simulink model "exp4M_CSVPosRefCtrl"  (R2020a)
settings: Solver=FixedStepAuto  StartTime=0.0  StopTime=20.0313  RelTol=1e-3
InitFcn:
  | %Motor1 = Epos4(1,0);
  | %Motor2 = Epos4(2,0);
  | load exp2MSetup sm_path1
model workspace (MAT data in the model file):
  Kd1 = 0
  Kd2 = 0
  Kd3 = 0
  Kd4 = 0
  Ki1 = 7.10897656468
  Ki2 = 7.11405369329
  Ki3 = 7.10867391424
  Ki4 = 7.10556368704
  Kp1 = 103.345225154
  Kp2 = 107.682383041
  Kp3 = 112.167183406
  Kp4 = 116.854342442
  N1 = 100
  N2 = 100
  N3 = 100
  N4 = 100
undefined symbols (not defined in the file or in its folder): x28_000006_reduction, x607325_PPR
libraries: simulink x4
CloseFcn:
  | %delete(Motor1);
  | %delete(Motor2);
settings Model: DataDictionary=MotorInfo.sldd  SimulationMode=accelerator  EnablePacing=on  OrderedModelArguments=off  Creator=khoi  LastModifiedBy=khoi
settings DataIOCC: InspectSignalLogs=on
settings RTWCC: GenCodeOnly=on

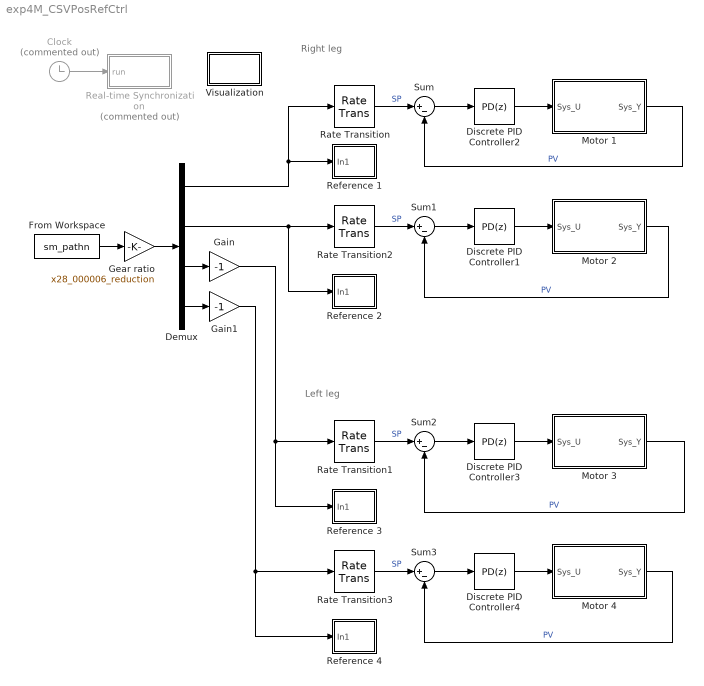
== system exp4M_CSVPosRefCtrl ==
  note: Right leg
  note: Left leg
  Clock : Clock  Commented=on
  Demux : Demux
  Discrete PID Controller1 : simulink/Continuous/PID Controller  Controller=PD  Form=Parallel  TimeDomain=Discrete-time  UseExternalTs=off  SampleTime=-1  IntegratorMethod=Forward Euler  FilterMethod=Forward Euler  ControllerParametersSource=internal  P=Kp2  I=Ki2  D=Kd2  UseFilter=on  N=N2  TunerSelectOption=Transfer Function Based (PID Tuner App)  InitialConditionSource=internal  InitialConditionForIntegrator=0  InitialConditionForFilter=0  DifferentiatorICPrevScaledInput=0  ExternalReset=none  TrackingMode=off  Kt=1  LimitOutput=off  UpperSaturationLimit=2000  LowerSaturationLimit=-2000  LinearizeAsGain=off  AntiWindupMode=clamping  Kb=1  POutMin=[]  POutMax=[]  IOutMin=[]  IOutMax=[]  DOutMin=[]  DOutMax=[]  NOutMin=[]  NOutMax=[]  SumOutMin=[]  SumOutMax=[]  SaturationOutMin=[]  SaturationOutMax=[]  PParamMin=[]  PParamMax=[]  IParamMin=[]  IParamMax=[]  DParamMin=[]  DParamMax=[]  NParamMin=[]  NParamMax=[]  KbParamMin=[]  KbParamMax=[]  KtParamMin=[]  KtParamMax=[]  KbOutMin=[]  KbOutMax=[]  KtOutMin=[]  KtOutMax=[]  IntegratorOutMin=[]  IntegratorOutMax=[]  FilterOutMin=[]  FilterOutMax=[]  SumI1OutMin=[]  SumI1OutMax=[]  SumI2OutMin=[]  SumI2OutMax=[]  SumI3OutMin=[]  SumI3OutMax=[]  SumI4OutMin=[]  SumI4OutMax=[]  SumDOutMin=[]  SumDOutMax=[]  DifferentiatorOutMin=[]  DifferentiatorOutMax=[]  FilterDiffOutCoefMin=[]  FilterDiffOutCoefMax=[]  ReciprocalOutMin=[]  ReciprocalOutMax=[]  SumDenOutMin=[]  SumDenOutMax=[]  SumNumOutMin=[]  SumNumOutMax=[]  DivideOutMin=[]  DivideOutMax=[]  UdiffTsProdOutMin=[]  UdiffTsProdOutMax=[]  NTsProdOutMin=[]  NTsProdOutMax=[]  UintegralTsProdOutMin=[]  UintegralTsProdOutMax=[]  UngainTsProdOutMin=[]  UngainTsProdOutMax=[]  IntegratorContinuousStateAttributes=''  IntegratorStateMustResolveToSignalObject=off  IntegratorRTWStateStorageClass=Auto  FilterContinuousStateAttributes=''  FilterStateMustResolveToSignalObject=off  FilterRTWStateStorageClass=Auto  ParallelPVariant=InternalParameters  IdealPVariant=Disabled  IVariant=Disabled  DVariant=InternalParameters  IntegratorVariant=Disabled  SatVariant=Disabled  AWVariant=Disabled  PCopyVariant=Disabled  TRVariant=Disabled  FdbkBlocksVariant=Forward  IdealPFdbkVariant=Disabled  SatFdbkVariant=Disabled  DerivativeFilterVariant=ForwardEulerFilter  NVariant=InternalParameters  NCopyVariant=Disabled  FilterICVariant=InternalICsFilter  IntegratorICVariant=Disabled  ExternalResetVariant=Disabled  TRSumVariant=Passthrough  SumFdbkVariant=Disabled  SumVariant=Sum_PD  TsampFilterVariant=InternalTs  TsampNgainVariant=Passthrough  TsampIntegralVariant=Disabled_SignalSpec
  Discrete PID Controller2 : simulink/Continuous/PID Controller  Controller=PD  Form=Parallel  TimeDomain=Discrete-time  UseExternalTs=off  SampleTime=-1  IntegratorMethod=Forward Euler  FilterMethod=Forward Euler  ControllerParametersSource=internal  P=Kp1  I=Ki1  D=Kd1  UseFilter=on  N=N1  TunerSelectOption=Transfer Function Based (PID Tuner App)  InitialConditionSource=internal  InitialConditionForIntegrator=0  InitialConditionForFilter=0  DifferentiatorICPrevScaledInput=0  ExternalReset=none  TrackingMode=off  Kt=1  LimitOutput=off  UpperSaturationLimit=2000  LowerSaturationLimit=-2000  LinearizeAsGain=off  AntiWindupMode=clamping  Kb=1  POutMin=[]  POutMax=[]  IOutMin=[]  IOutMax=[]  DOutMin=[]  DOutMax=[]  NOutMin=[]  NOutMax=[]  SumOutMin=[]  SumOutMax=[]  SaturationOutMin=[]  SaturationOutMax=[]  PParamMin=[]  PParamMax=[]  IParamMin=[]  IParamMax=[]  DParamMin=[]  DParamMax=[]  NParamMin=[]  NParamMax=[]  KbParamMin=[]  KbParamMax=[]  KtParamMin=[]  KtParamMax=[]  KbOutMin=[]  KbOutMax=[]  KtOutMin=[]  KtOutMax=[]  IntegratorOutMin=[]  IntegratorOutMax=[]  FilterOutMin=[]  FilterOutMax=[]  SumI1OutMin=[]  SumI1OutMax=[]  SumI2OutMin=[]  SumI2OutMax=[]  SumI3OutMin=[]  SumI3OutMax=[]  SumI4OutMin=[]  SumI4OutMax=[]  SumDOutMin=[]  SumDOutMax=[]  DifferentiatorOutMin=[]  DifferentiatorOutMax=[]  FilterDiffOutCoefMin=[]  FilterDiffOutCoefMax=[]  ReciprocalOutMin=[]  ReciprocalOutMax=[]  SumDenOutMin=[]  SumDenOutMax=[]  SumNumOutMin=[]  SumNumOutMax=[]  DivideOutMin=[]  DivideOutMax=[]  UdiffTsProdOutMin=[]  UdiffTsProdOutMax=[]  NTsProdOutMin=[]  NTsProdOutMax=[]  UintegralTsProdOutMin=[]  UintegralTsProdOutMax=[]  UngainTsProdOutMin=[]  UngainTsProdOutMax=[]  IntegratorContinuousStateAttributes=''  IntegratorStateMustResolveToSignalObject=off  IntegratorRTWStateStorageClass=Auto  FilterContinuousStateAttributes=''  FilterStateMustResolveToSignalObject=off  FilterRTWStateStorageClass=Auto  ParallelPVariant=InternalParameters  IdealPVariant=Disabled  IVariant=Disabled  DVariant=InternalParameters  IntegratorVariant=Disabled  SatVariant=Disabled  AWVariant=Disabled  PCopyVariant=Disabled  TRVariant=Disabled  FdbkBlocksVariant=Forward  IdealPFdbkVariant=Disabled  SatFdbkVariant=Disabled  DerivativeFilterVariant=ForwardEulerFilter  NVariant=InternalParameters  NCopyVariant=Disabled  FilterICVariant=InternalICsFilter  IntegratorICVariant=Disabled  ExternalResetVariant=Disabled  TRSumVariant=Passthrough  SumFdbkVariant=Disabled  SumVariant=Sum_PD  TsampFilterVariant=InternalTs  TsampNgainVariant=Passthrough  TsampIntegralVariant=Disabled_SignalSpec
  Discrete PID Controller3 : simulink/Continuous/PID Controller  Controller=PD  Form=Parallel  TimeDomain=Discrete-time  UseExternalTs=off  SampleTime=-1  IntegratorMethod=Forward Euler  FilterMethod=Forward Euler  ControllerParametersSource=internal  P=Kp3  I=Ki3  D=Kd3  UseFilter=on  N=N3  TunerSelectOption=Transfer Function Based (PID Tuner App)  InitialConditionSource=internal  InitialConditionForIntegrator=0  InitialConditionForFilter=0  DifferentiatorICPrevScaledInput=0  ExternalReset=none  TrackingMode=off  Kt=1  LimitOutput=off  UpperSaturationLimit=2000  LowerSaturationLimit=-2000  LinearizeAsGain=off  AntiWindupMode=clamping  Kb=1  POutMin=[]  POutMax=[]  IOutMin=[]  IOutMax=[]  DOutMin=[]  DOutMax=[]  NOutMin=[]  NOutMax=[]  SumOutMin=[]  SumOutMax=[]  SaturationOutMin=[]  SaturationOutMax=[]  PParamMin=[]  PParamMax=[]  IParamMin=[]  IParamMax=[]  DParamMin=[]  DParamMax=[]  NParamMin=[]  NParamMax=[]  KbParamMin=[]  KbParamMax=[]  KtParamMin=[]  KtParamMax=[]  KbOutMin=[]  KbOutMax=[]  KtOutMin=[]  KtOutMax=[]  IntegratorOutMin=[]  IntegratorOutMax=[]  FilterOutMin=[]  FilterOutMax=[]  SumI1OutMin=[]  SumI1OutMax=[]  SumI2OutMin=[]  SumI2OutMax=[]  SumI3OutMin=[]  SumI3OutMax=[]  SumI4OutMin=[]  SumI4OutMax=[]  SumDOutMin=[]  SumDOutMax=[]  DifferentiatorOutMin=[]  DifferentiatorOutMax=[]  FilterDiffOutCoefMin=[]  FilterDiffOutCoefMax=[]  ReciprocalOutMin=[]  ReciprocalOutMax=[]  SumDenOutMin=[]  SumDenOutMax=[]  SumNumOutMin=[]  SumNumOutMax=[]  DivideOutMin=[]  DivideOutMax=[]  UdiffTsProdOutMin=[]  UdiffTsProdOutMax=[]  NTsProdOutMin=[]  NTsProdOutMax=[]  UintegralTsProdOutMin=[]  UintegralTsProdOutMax=[]  UngainTsProdOutMin=[]  UngainTsProdOutMax=[]  IntegratorContinuousStateAttributes=''  IntegratorStateMustResolveToSignalObject=off  IntegratorRTWStateStorageClass=Auto  FilterContinuousStateAttributes=''  FilterStateMustResolveToSignalObject=off  FilterRTWStateStorageClass=Auto  ParallelPVariant=InternalParameters  IdealPVariant=Disabled  IVariant=Disabled  DVariant=InternalParameters  IntegratorVariant=Disabled  SatVariant=Disabled  AWVariant=Disabled  PCopyVariant=Disabled  TRVariant=Disabled  FdbkBlocksVariant=Forward  IdealPFdbkVariant=Disabled  SatFdbkVariant=Disabled  DerivativeFilterVariant=ForwardEulerFilter  NVariant=InternalParameters  NCopyVariant=Disabled  FilterICVariant=InternalICsFilter  IntegratorICVariant=Disabled  ExternalResetVariant=Disabled  TRSumVariant=Passthrough  SumFdbkVariant=Disabled  SumVariant=Sum_PD  TsampFilterVariant=InternalTs  TsampNgainVariant=Passthrough  TsampIntegralVariant=Disabled_SignalSpec
  Discrete PID Controller4 : simulink/Continuous/PID Controller  Controller=PD  Form=Parallel  TimeDomain=Discrete-time  UseExternalTs=off  SampleTime=-1  IntegratorMethod=Forward Euler  FilterMethod=Forward Euler  ControllerParametersSource=internal  P=Kp4  I=Ki4  D=Kd4  UseFilter=on  N=N4  TunerSelectOption=Transfer Function Based (PID Tuner App)  InitialConditionSource=internal  InitialConditionForIntegrator=0  InitialConditionForFilter=0  DifferentiatorICPrevScaledInput=0  ExternalReset=none  TrackingMode=off  Kt=1  LimitOutput=off  UpperSaturationLimit=2000  LowerSaturationLimit=-2000  LinearizeAsGain=off  AntiWindupMode=clamping  Kb=1  POutMin=[]  POutMax=[]  IOutMin=[]  IOutMax=[]  DOutMin=[]  DOutMax=[]  NOutMin=[]  NOutMax=[]  SumOutMin=[]  SumOutMax=[]  SaturationOutMin=[]  SaturationOutMax=[]  PParamMin=[]  PParamMax=[]  IParamMin=[]  IParamMax=[]  DParamMin=[]  DParamMax=[]  NParamMin=[]  NParamMax=[]  KbParamMin=[]  KbParamMax=[]  KtParamMin=[]  KtParamMax=[]  KbOutMin=[]  KbOutMax=[]  KtOutMin=[]  KtOutMax=[]  IntegratorOutMin=[]  IntegratorOutMax=[]  FilterOutMin=[]  FilterOutMax=[]  SumI1OutMin=[]  SumI1OutMax=[]  SumI2OutMin=[]  SumI2OutMax=[]  SumI3OutMin=[]  SumI3OutMax=[]  SumI4OutMin=[]  SumI4OutMax=[]  SumDOutMin=[]  SumDOutMax=[]  DifferentiatorOutMin=[]  DifferentiatorOutMax=[]  FilterDiffOutCoefMin=[]  FilterDiffOutCoefMax=[]  ReciprocalOutMin=[]  ReciprocalOutMax=[]  SumDenOutMin=[]  SumDenOutMax=[]  SumNumOutMin=[]  SumNumOutMax=[]  DivideOutMin=[]  DivideOutMax=[]  UdiffTsProdOutMin=[]  UdiffTsProdOutMax=[]  NTsProdOutMin=[]  NTsProdOutMax=[]  UintegralTsProdOutMin=[]  UintegralTsProdOutMax=[]  UngainTsProdOutMin=[]  UngainTsProdOutMax=[]  IntegratorContinuousStateAttributes=''  IntegratorStateMustResolveToSignalObject=off  IntegratorRTWStateStorageClass=Auto  FilterContinuousStateAttributes=''  FilterStateMustResolveToSignalObject=off  FilterRTWStateStorageClass=Auto  ParallelPVariant=InternalParameters  IdealPVariant=Disabled  IVariant=Disabled  DVariant=InternalParameters  IntegratorVariant=Disabled  SatVariant=Disabled  AWVariant=Disabled  PCopyVariant=Disabled  TRVariant=Disabled  FdbkBlocksVariant=Forward  IdealPFdbkVariant=Disabled  SatFdbkVariant=Disabled  DerivativeFilterVariant=ForwardEulerFilter  NVariant=InternalParameters  NCopyVariant=Disabled  FilterICVariant=InternalICsFilter  IntegratorICVariant=Disabled  ExternalResetVariant=Disabled  TRSumVariant=Passthrough  SumFdbkVariant=Disabled  SumVariant=Sum_PD  TsampFilterVariant=InternalTs  TsampNgainVariant=Passthrough  TsampIntegralVariant=Disabled_SignalSpec
  From Workspace : FromWorkspace  VariableName=sm_pathn  SampleTime=0.01
  Gain : Gain  Gain=-1
  Gain1 : Gain  Gain=-1
  Gear ratio : Gain  Gain=x28_000006_reduction
  Motor 1 : Subsystem
  Motor 2 : Subsystem
  Motor 3 : Subsystem
  Motor 4 : Subsystem
  Rate Transition{,1..3} (4 alike) : RateTransition  OutPortSampleTime=0.02
  Real-time Synchronization : Subsystem  Commented=on
  Reference 1 : Subsystem
  Reference 2 : Subsystem
  Reference 3 : Subsystem
  Reference 4 : Subsystem
  Sum{,1..3} (4 alike) : Sum  Inputs=|+-
  Visualization : Subsystem
  wires:
  Clock/1 -> Real-time Synchronization/1(run)
  Demux/1 -> Rate Transition/1, Reference 1/1(In1)
  Sum/1 -> Discrete PID Controller2/1
  Sum1/1 -> Discrete PID Controller1/1
  From Workspace/1 -> Gear ratio/1
  Demux/2 -> Reference 2/1(In1), Rate Transition2/1
  Gear ratio/1 -> Demux/1
  Rate Transition/1 -> Sum/1  "SP"
  Discrete PID Controller2/1 -> Motor 1/1(Sys_U)
  Motor 1/1(Sys_Y) -> Sum/2  "PV"
  Discrete PID Controller1/1 -> Motor 2/1(Sys_U)
  Rate Transition2/1 -> Sum1/1  "SP"
  Rate Transition1/1 -> Sum2/1  "SP"
  Motor 3/1(Sys_Y) -> Sum2/2  "PV"
  Discrete PID Controller3/1 -> Motor 3/1(Sys_U)
  Sum2/1 -> Discrete PID Controller3/1
  Sum3/1 -> Discrete PID Controller4/1
  Discrete PID Controller4/1 -> Motor 4/1(Sys_U)
  Motor 4/1(Sys_Y) -> Sum3/2  "PV"
  Rate Transition3/1 -> Sum3/1  "SP"
  Demux/3 -> Gain/1
  Demux/4 -> Gain1/1
  Gain/1 -> Rate Transition1/1, Reference 3/1(In1)
  Gain1/1 -> Reference 4/1(In1), Rate Transition3/1
  Motor 2/1(Sys_Y) -> Sum1/2  "PV"

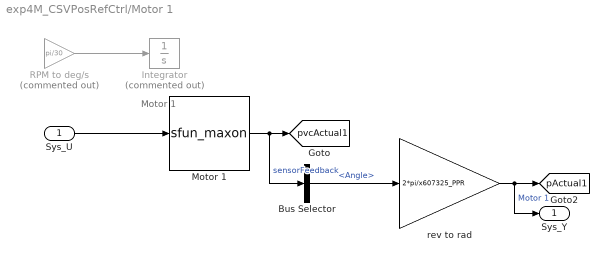
== system exp4M_CSVPosRefCtrl/Motor 1 ==
  note: Motor 1
  Sys_U : Inport
  Bus Selector : BusSelector  OutputSignals=Angle
  Integrator : Integrator  Commented=on
  Motor 1 : S-Function  FunctionName=sfun_maxon  Parameters=NodeID, DeltaT, OpMode  SFunctionDeploymentMode=off  EnableBusSupport=off  mask{NodeID=1, DeltaT=0.2, OpMode=Cyclic synchronous velocity mode, P_cur=0, I_cur=0, P_pos=0, I_pos=0, D_pos=0, v_posGainFF=0, a_posGainFF=0, P_vel=0, I_vel=0, v_velGainFF=0, a_velGainFF=0, f_velCutoff=0}
      mask prompts: NodeID "Node ID"; DeltaT "Sample time (s)"; OpMode "Operation mode"; P_cur "P gain"; I_cur "I gain"; P_pos "P gain"; I_pos "I gain"; D_pos "D gain"; v_posGainFF "FF velocity gain"; a_posGainFF "FF acceleration gain"; P_vel "P gain"; I_vel "I gain"; v_velGainFF "Feed-forward velocity gain"; a_velGainFF "Feed-forward acceleration gain"; f_velCutoff "Filter cut-off frequency"
      mask TypeOptions OpMode: Cyclic synchronous current (torque) mode | Cyclic synchronous velocity mode | Cyclic synchronous position mode | Profile velocity mode | Profile position mode
      mask DialogControl DescGroupVar Prompt: Motor Parameters
      mask DialogControl DescTextVar Prompt: The block outputs MotorInfo bus signal, which consists of the following variables: angle (increment), speed (rpm), current (mA)
      mask DialogControl Container6 Prompt: Motor
      mask DialogControl Container14 Prompt: Controller Parameters
      mask DialogControl DescTextVar_copy Prompt: This tab is experimental and does not implemented yet. Changing these parameters will not affect the motor performance.
      mask DialogControl Container15 Prompt: Current controller parameter set
      mask DialogControl Container15_copy Prompt: Position controller parameter set
      mask DialogControl Container15_copy_copy Prompt: Velocity controller parameter set
      mask Display:
      | disp('Maxon motor\nHIL');
      | % port_label('input', 1, 'inputSignal');
      | % port_label('output', 1, 'SENSR');
  RPM to deg/s : Gain  Commented=on  Gain=pi/30
  rev to rad : Gain  Gain=2*pi/x607325_PPR
  Sys_Y : Outport
  tag scope: pActual1=global, pvcActual1=global
  wires:
  Motor 1/1 -> [pvcActual1], Bus Selector/1  "sensorFeedback"
  rev to rad/1 -> Sys_Y/1, [pActual1]  "Motor 1"
  Sys_U/1 -> Motor 1/1
  RPM to deg/s/1 -> Integrator/1
  Bus Selector/1 -> rev to rad/1  "<Angle>"

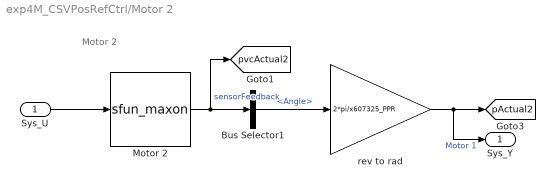
== system exp4M_CSVPosRefCtrl/Motor 2 ==
  note: Motor 2
  Sys_U : Inport
  Bus Selector1 : BusSelector  OutputSignals=Angle
  Motor 2 : S-Function  FunctionName=sfun_maxon  Parameters=NodeID, DeltaT, OpMode  SFunctionDeploymentMode=off  EnableBusSupport=off  mask{NodeID=2, DeltaT=0.2, OpMode=Cyclic synchronous velocity mode, P_cur=0, I_cur=0, P_pos=0, I_pos=0, D_pos=0, v_posGainFF=0, a_posGainFF=0, P_vel=0, I_vel=0, v_velGainFF=0, a_velGainFF=0, f_velCutoff=0}
      mask prompts: NodeID "Node ID"; DeltaT "Sample time (s)"; OpMode "Operation mode"; P_cur "P gain"; I_cur "I gain"; P_pos "P gain"; I_pos "I gain"; D_pos "D gain"; v_posGainFF "FF velocity gain"; a_posGainFF "FF acceleration gain"; P_vel "P gain"; I_vel "I gain"; v_velGainFF "Feed-forward velocity gain"; a_velGainFF "Feed-forward acceleration gain"; f_velCutoff "Filter cut-off frequency"
      mask TypeOptions OpMode: Cyclic synchronous current (torque) mode | Cyclic synchronous velocity mode | Cyclic synchronous position mode | Profile velocity mode | Profile position mode
      mask DialogControl DescGroupVar Prompt: Motor Parameters
      mask DialogControl DescTextVar Prompt: The block outputs MotorInfo bus signal, which consists of the following variables: angle (increment), speed (rpm), current (mA)
      mask DialogControl Container6 Prompt: Motor
      mask DialogControl Container14 Prompt: Controller Parameters
      mask DialogControl DescTextVar_copy Prompt: This tab is experimental and does not implemented yet. Changing these parameters will not affect the motor performance.
      mask DialogControl Container15 Prompt: Current controller parameter set
      mask DialogControl Container15_copy Prompt: Position controller parameter set
      mask DialogControl Container15_copy_copy Prompt: Velocity controller parameter set
      mask Display:
      | disp('Maxon motor\nHIL');
      | % port_label('input', 1, 'inputSignal');
      | % port_label('output', 1, 'SENSR');
  rev to rad : Gain  Gain=2*pi/x607325_PPR
  Sys_Y : Outport
  tag scope: pActual2=global, pvcActual2=global
  wires:
  Bus Selector1/1 -> rev to rad/1  "<Angle>"
  Sys_U/1 -> Motor 2/1
  rev to rad/1 -> Sys_Y/1, [pActual2]  "Motor 1"
  Motor 2/1 -> [pvcActual2], Bus Selector1/1  "sensorFeedback"

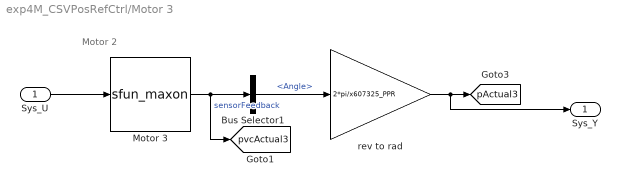
== system exp4M_CSVPosRefCtrl/Motor 3 ==
  note: Motor 2
  Sys_U : Inport
  Bus Selector1 : BusSelector  OutputSignals=Angle
  Motor 3 : S-Function  FunctionName=sfun_maxon  Parameters=NodeID, DeltaT, OpMode  SFunctionDeploymentMode=off  EnableBusSupport=off  mask{NodeID=3, DeltaT=0.2, OpMode=Cyclic synchronous velocity mode, P_cur=0, I_cur=0, P_pos=0, I_pos=0, D_pos=0, v_posGainFF=0, a_posGainFF=0, P_vel=0, I_vel=0, v_velGainFF=0, a_velGainFF=0, f_velCutoff=0}
      mask prompts: NodeID "Node ID"; DeltaT "Sample time (s)"; OpMode "Operation mode"; P_cur "P gain"; I_cur "I gain"; P_pos "P gain"; I_pos "I gain"; D_pos "D gain"; v_posGainFF "FF velocity gain"; a_posGainFF "FF acceleration gain"; P_vel "P gain"; I_vel "I gain"; v_velGainFF "Feed-forward velocity gain"; a_velGainFF "Feed-forward acceleration gain"; f_velCutoff "Filter cut-off frequency"
      mask TypeOptions OpMode: Cyclic synchronous current (torque) mode | Cyclic synchronous velocity mode | Cyclic synchronous position mode | Profile velocity mode | Profile position mode
      mask DialogControl DescGroupVar Prompt: Motor Parameters
      mask DialogControl DescTextVar Prompt: The block outputs MotorInfo bus signal, which consists of the following variables: angle (increment), speed (rpm), current (mA)
      mask DialogControl Container6 Prompt: Motor
      mask DialogControl Container14 Prompt: Controller Parameters
      mask DialogControl DescTextVar_copy Prompt: This tab is experimental and does not implemented yet. Changing these parameters will not affect the motor performance.
      mask DialogControl Container15 Prompt: Current controller parameter set
      mask DialogControl Container15_copy Prompt: Position controller parameter set
      mask DialogControl Container15_copy_copy Prompt: Velocity controller parameter set
      mask Display:
      | disp('Maxon motor\nHIL');
      | % port_label('input', 1, 'inputSignal');
      | % port_label('output', 1, 'SENSR');
  rev to rad : Gain  Gain=2*pi/x607325_PPR
  Sys_Y : Outport
  tag scope: pActual3=global, pvcActual3=global
  wires:
  Sys_U/1 -> Motor 3/1
  Bus Selector1/1 -> rev to rad/1  "<Angle>"
  rev to rad/1 -> Sys_Y/1, [pActual3]
  Motor 3/1 -> Bus Selector1/1, [pvcActual3]  "sensorFeedback"

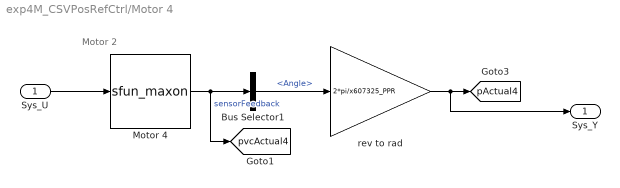
== system exp4M_CSVPosRefCtrl/Motor 4 ==
  note: Motor 2
  Sys_U : Inport
  Bus Selector1 : BusSelector  OutputSignals=Angle
  Motor 4 : S-Function  FunctionName=sfun_maxon  Parameters=NodeID, DeltaT, OpMode  SFunctionDeploymentMode=off  EnableBusSupport=off  mask{NodeID=4, DeltaT=0.2, OpMode=Cyclic synchronous velocity mode, P_cur=0, I_cur=0, P_pos=0, I_pos=0, D_pos=0, v_posGainFF=0, a_posGainFF=0, P_vel=0, I_vel=0, v_velGainFF=0, a_velGainFF=0, f_velCutoff=0}
      mask prompts: NodeID "Node ID"; DeltaT "Sample time (s)"; OpMode "Operation mode"; P_cur "P gain"; I_cur "I gain"; P_pos "P gain"; I_pos "I gain"; D_pos "D gain"; v_posGainFF "FF velocity gain"; a_posGainFF "FF acceleration gain"; P_vel "P gain"; I_vel "I gain"; v_velGainFF "Feed-forward velocity gain"; a_velGainFF "Feed-forward acceleration gain"; f_velCutoff "Filter cut-off frequency"
      mask TypeOptions OpMode: Cyclic synchronous current (torque) mode | Cyclic synchronous velocity mode | Cyclic synchronous position mode | Profile velocity mode | Profile position mode
      mask DialogControl DescGroupVar Prompt: Motor Parameters
      mask DialogControl DescTextVar Prompt: The block outputs MotorInfo bus signal, which consists of the following variables: angle (increment), speed (rpm), current (mA)
      mask DialogControl Container6 Prompt: Motor
      mask DialogControl Container14 Prompt: Controller Parameters
      mask DialogControl DescTextVar_copy Prompt: This tab is experimental and does not implemented yet. Changing these parameters will not affect the motor performance.
      mask DialogControl Container15 Prompt: Current controller parameter set
      mask DialogControl Container15_copy Prompt: Position controller parameter set
      mask DialogControl Container15_copy_copy Prompt: Velocity controller parameter set
      mask Display:
      | disp('Maxon motor\nHIL');
      | % port_label('input', 1, 'inputSignal');
      | % port_label('output', 1, 'SENSR');
  rev to rad : Gain  Gain=2*pi/x607325_PPR
  Sys_Y : Outport
  tag scope: pActual4=global, pvcActual4=global
  wires:
  Sys_U/1 -> Motor 4/1
  Bus Selector1/1 -> rev to rad/1  "<Angle>"
  rev to rad/1 -> Sys_Y/1, [pActual4]
  Motor 4/1 -> [pvcActual4], Bus Selector1/1  "sensorFeedback"

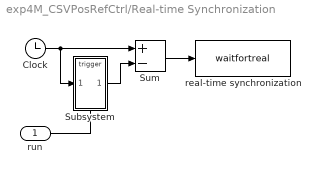
== system exp4M_CSVPosRefCtrl/Real-time Synchronization ==
  run : Inport
  Clock : Clock
  Subsystem : Subsystem  TreatAsAtomicUnit=on
  Sum : Sum  Inputs=+-  InputSameDT=on  SaturateOnIntegerOverflow=on  OutDataTypeStr=Inherit: Same as first input
  real-time synchronization : MATLABFcn  MATLABFcn=waitfortreal  OutputDimensions=0
  wires:
  Clock/1 -> Subsystem/1(In), Sum/1
  Subsystem/1(Out) -> Sum/2
  Sum/1 -> real-time synchronization/1
  run/1 -> Subsystem/Trigger

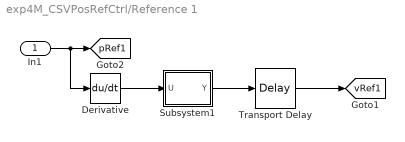
== system exp4M_CSVPosRefCtrl/Reference 1 ==
  In1 : Inport
  Derivative : Derivative
  Subsystem1 : Subsystem
      mask Display: disp('To rpm')
  Transport Delay : TransportDelay  DelayTime=0.1
  tag scope: pRef1=global, vRef1=global
  wires:
  Subsystem1/1(Y) -> Transport Delay/1
  Derivative/1 -> Subsystem1/1(U)
  In1/1 -> Derivative/1, [pRef1]
  Transport Delay/1 -> [vRef1]

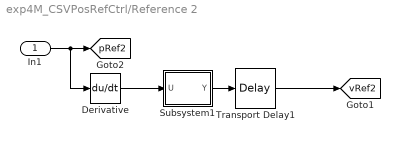
== system exp4M_CSVPosRefCtrl/Reference 2 ==
  In1 : Inport
  Derivative : Derivative
  Subsystem1 : Subsystem
      mask Display: disp('To rpm')
  Transport Delay1 : TransportDelay  DelayTime=0.1
  tag scope: pRef2=global, vRef2=global
  wires:
  Subsystem1/1(Y) -> Transport Delay1/1
  In1/1 -> [pRef2], Derivative/1
  Derivative/1 -> Subsystem1/1(U)
  Transport Delay1/1 -> [vRef2]

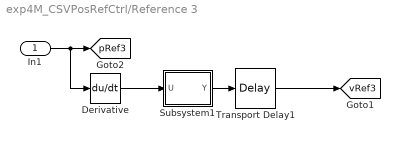
== system exp4M_CSVPosRefCtrl/Reference 3 ==
  In1 : Inport
  Derivative : Derivative
  Subsystem1 : Subsystem
      mask Display: disp('To rpm')
  Transport Delay1 : TransportDelay  DelayTime=0.1
  tag scope: pRef3=global, vRef3=global
  wires:
  Transport Delay1/1 -> [vRef3]
  Derivative/1 -> Subsystem1/1(U)
  In1/1 -> Derivative/1, [pRef3]
  Subsystem1/1(Y) -> Transport Delay1/1

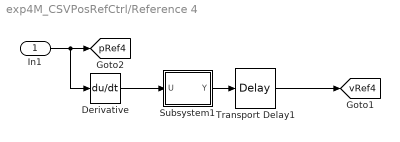
== system exp4M_CSVPosRefCtrl/Reference 4 ==
  In1 : Inport
  Derivative : Derivative
  Subsystem1 : Subsystem
      mask Display: disp('To rpm')
  Transport Delay1 : TransportDelay  DelayTime=0.1
  tag scope: pRef4=global, vRef4=global
  wires:
  Subsystem1/1(Y) -> Transport Delay1/1
  In1/1 -> [pRef4], Derivative/1
  Derivative/1 -> Subsystem1/1(U)
  Transport Delay1/1 -> [vRef4]

== system exp4M_CSVPosRefCtrl/Visualization ==
  Left leg : Subsystem
  Right leg : Subsystem
  current : Scope  NumInputPorts=2
  position : Scope  NumInputPorts=2
  speed : Scope  NumInputPorts=2
  wires:
  Right leg/3(Out4) -> current/2
  Left leg/1(Out1) -> position/1
  Left leg/2(Out2) -> speed/1
  Right leg/2(Out1) -> speed/2
  Left leg/3(Out4) -> current/1
  Right leg/1(Out2) -> position/2

== system exp4M_CSVPosRefCtrl/Real-time Synchronization/Subsystem ==
  In : Inport
  Trigger : TriggerPort  VariantControl=(inherit)
  Out : Outport  InitialOutput=0
  wires:
  In/1 -> Out/1

== system exp4M_CSVPosRefCtrl/Reference 1/Subsystem1 ==
  U : Inport
  rad/s to rpm : Gain  Gain=60/(2*pi)
  Y : Outport
  wires:
  rad/s to rpm/1 -> Y/1
  U/1 -> rad/s to rpm/1

== system exp4M_CSVPosRefCtrl/Reference 2/Subsystem1 ==
  U : Inport
  rad/s to rpm : Gain  Gain=60/(2*pi)
  Y : Outport
  wires:
  rad/s to rpm/1 -> Y/1
  U/1 -> rad/s to rpm/1

== system exp4M_CSVPosRefCtrl/Reference 3/Subsystem1 ==
  U : Inport
  rad/s to rpm : Gain  Gain=60/(2*pi)
  Y : Outport
  wires:
  U/1 -> rad/s to rpm/1
  rad/s to rpm/1 -> Y/1

== system exp4M_CSVPosRefCtrl/Reference 4/Subsystem1 ==
  U : Inport
  rad/s to rpm : Gain  Gain=60/(2*pi)
  Y : Outport
  wires:
  rad/s to rpm/1 -> Y/1
  U/1 -> rad/s to rpm/1

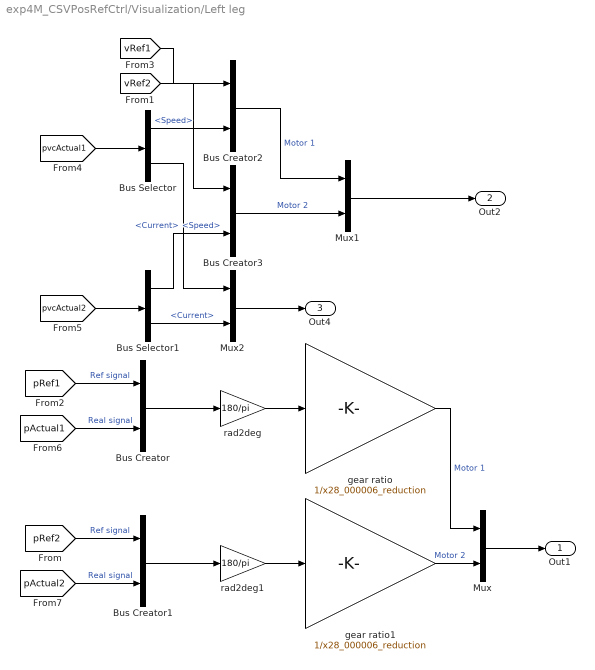
== system exp4M_CSVPosRefCtrl/Visualization/Left leg ==
  Bus Selector : BusSelector  OutputSignals=Speed,Current
  Bus Selector1 : BusSelector  OutputSignals=Speed,Current
  Bus Creator{,1..3} (4 alike) : BusCreator  Inputs=2
  Mux : Mux  Inputs=2
  Mux1 : Mux  Inputs=2
  Mux2 : Mux  Inputs=2
  gear ratio : Gain  Gain=1/x28_000006_reduction
  gear ratio1 : Gain  Gain=1/x28_000006_reduction
  rad2deg : Gain  Gain=180/pi
  rad2deg1 : Gain  Gain=180/pi
  Out1 : Outport
  Out2 : Outport  Port=2
  Out4 : Outport  Port=3
  wires:
  [pRef1] -> Bus Creator/1  "Ref signal"
  rad2deg1/1 -> gear ratio1/1
  [vRef2] -> Bus Creator3/1
  Mux/1 -> Out1/1
  [pActual2] -> Bus Creator1/2  "Real signal"
  [pRef2] -> Bus Creator1/1  "Ref signal"
  [vRef1] -> Bus Creator2/1
  rad2deg/1 -> gear ratio/1
  [pvcActual2] -> Bus Selector1/1
  Bus Creator3/1 -> Mux1/2  "Motor 2"
  Mux2/1 -> Out4/1
  Bus Selector1/1 -> Bus Creator3/2  "<Speed>"
  [pActual1] -> Bus Creator/2  "Real signal"
  Bus Creator1/1 -> rad2deg1/1
  Bus Creator/1 -> rad2deg/1
  gear ratio1/1 -> Mux/2  "Motor 2"
  Bus Selector/1 -> Bus Creator2/2  "<Speed>"
  Bus Selector1/2 -> Mux2/2  "<Current>"
  Bus Creator2/1 -> Mux1/1  "Motor 1"
  Bus Selector/2 -> Mux2/1  "<Current>"
  Mux1/1 -> Out2/1
  [pvcActual1] -> Bus Selector/1
  gear ratio/1 -> Mux/1  "Motor 1"

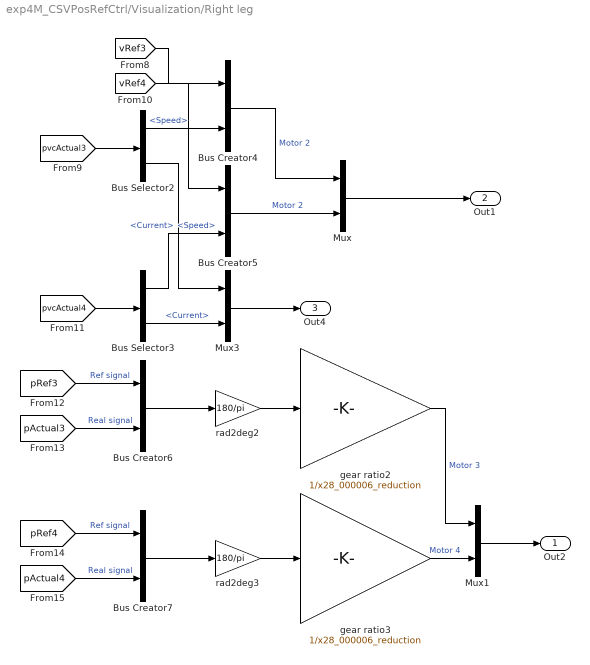
== system exp4M_CSVPosRefCtrl/Visualization/Right leg ==
  Bus Selector2 : BusSelector  OutputSignals=Speed,Current
  Bus Selector3 : BusSelector  OutputSignals=Speed,Current
  Bus Creator{4..7} (4 alike) : BusCreator  Inputs=2
  Mux : Mux  Inputs=2
  Mux1 : Mux  Inputs=2
  Mux3 : Mux  Inputs=2
  gear ratio2 : Gain  Gain=1/x28_000006_reduction
  gear ratio3 : Gain  Gain=1/x28_000006_reduction
  rad2deg2 : Gain  Gain=180/pi
  rad2deg3 : Gain  Gain=180/pi
  Out2 : Outport
  Out1 : Outport  Port=2
  Out4 : Outport  Port=3
  wires:
  [pvcActual3] -> Bus Selector2/1
  [pRef4] -> Bus Creator7/1  "Ref signal"
  Bus Creator6/1 -> rad2deg2/1
  [pActual3] -> Bus Creator6/2  "Real signal"
  [pvcActual4] -> Bus Selector3/1
  rad2deg2/1 -> gear ratio2/1
  Bus Creator7/1 -> rad2deg3/1
  Bus Creator5/1 -> Mux/2  "Motor 2"
  Mux1/1 -> Out2/1
  Mux3/1 -> Out4/1
  Bus Selector2/1 -> Bus Creator4/2  "<Speed>"
  Bus Selector3/2 -> Mux3/2  "<Current>"
  [pRef3] -> Bus Creator6/1  "Ref signal"
  Bus Creator4/1 -> Mux/1  "Motor 2"
  rad2deg3/1 -> gear ratio3/1
  Bus Selector2/2 -> Mux3/1  "<Current>"
  [pActual4] -> Bus Creator7/2  "Real signal"
  Bus Selector3/1 -> Bus Creator5/2  "<Speed>"
  gear ratio3/1 -> Mux1/2  "Motor 4"
  gear ratio2/1 -> Mux1/1  "Motor 3"
  [vRef3] -> Bus Creator4/1
  [vRef4] -> Bus Creator5/1
  Mux/1 -> Out1/1
